simulink model "Model_14Bus_Microgrid_R2017b"  (R2017b)
settings: Solver=ode23tb  StartTime=0.0  StopTime=0.35  MaxStep=1e-2  RelTol=1e-3
InitFcn:
  | Set_parameters_R2018
StopFcn:
  | Save_Data;
  | Graphics;
values from neighbouring files (symbols this model uses):
  Clink = Ceq*2    (= 0.217013888889)    [Set_parameters_R2017b.m]    (also in Set_parameters_R2018.m)
  dis1 = 0.15    [Set_parameters_R2017b.m]    (also in Set_parameters_R2018.m)
  dis10 = 6    [Set_parameters_R2017b.m]    (also in Set_parameters_R2018.m)
  dis11 = 3    [Set_parameters_R2017b.m]    (also in Set_parameters_R2018.m)
  dis12 = 6    [Set_parameters_R2017b.m]    (also in Set_parameters_R2018.m)
  dis13 = 3    [Set_parameters_R2017b.m]    (also in Set_parameters_R2018.m)
  dis14 = 2    [Set_parameters_R2017b.m]    (also in Set_parameters_R2018.m)
  dis2 = 0.2    [Set_parameters_R2017b.m]    (also in Set_parameters_R2018.m)
  dis3 = 0.15    [Set_parameters_R2017b.m]    (also in Set_parameters_R2018.m)
  dis4 = 0.4    [Set_parameters_R2017b.m]    (also in Set_parameters_R2018.m)
  dis5 = 0.4    [Set_parameters_R2017b.m]    (also in Set_parameters_R2018.m)
  dis6 = 0.4    [Set_parameters_R2017b.m]    (also in Set_parameters_R2018.m)
  dis7 = 0.1    [Set_parameters_R2017b.m]    (also in Set_parameters_R2018.m)
  dis8 = 2    [Set_parameters_R2017b.m]    (also in Set_parameters_R2018.m)
  dis9 = 6    [Set_parameters_R2017b.m]    (also in Set_parameters_R2018.m)
  Fc = 33 * Fnom    (= 1980)    [Set_parameters_R2017b.m]    (also in Set_parameters_R2018.m)
  Fnom = 60    [Main_DC_MG.m]    (also in Set_parameters_R2017b.m; Set_parameters_R2018.m)
  Increment_MPPT = 0.01    [Set_parameters_R2017b.m]    (also in Set_parameters_R2018.m)
  Ki_Ireg = 20    [Set_parameters_R2017b.m]    (also in Set_parameters_R2018.m)
  Ki_VDCreg = 400    [Set_parameters_R2017b.m]    (also in Set_parameters_R2018.m)
  Kp_Ireg = 0.3    [Set_parameters_R2017b.m]    (also in Set_parameters_R2018.m)
  Kp_VDCreg = 2    [Set_parameters_R2017b.m]    (also in Set_parameters_R2018.m)
  LimitL_Ireg = -1.5    [Set_parameters_R2017b.m]    (also in Set_parameters_R2018.m)
  LimitL_VDCreg = -1.5    [Set_parameters_R2017b.m]    (also in Set_parameters_R2018.m)
  Limits_MPPT = [ 583 357 ]    [Set_parameters_R2017b.m]    (also in Set_parameters_R2018.m)
  LimitU_Ireg = 1.5    [Set_parameters_R2017b.m]    (also in Set_parameters_R2018.m)
  LimitU_VDCreg = 1.5    [Set_parameters_R2017b.m]    (also in Set_parameters_R2018.m)
  P_Load_2 = S_Load_2* PF_Load_2    (= 36000)    [Set_parameters_R2017b.m]    (also in Set_parameters_R2018.m)
  P_Load_3 = S_Load_3* PF_Load_3    (= 25500)    [Set_parameters_R2017b.m]    (also in Set_parameters_R2018.m)
  Pnom = 1e6    (= 1000000)    [Set_parameters_R2017b.m]    (also in Set_parameters_R2018.m)
  Pnom_T1 = 1.5e6    (= 1500000)    [Set_parameters_R2017b.m]    (also in Set_parameters_R2018.m)
  Pnom_T2 = 1.5e6    (= 1500000)    [Set_parameters_R2017b.m]    (also in Set_parameters_R2018.m)
  Pnom_T3 = 4e6    (= 4000000)    [Set_parameters_R2017b.m]    (also in Set_parameters_R2018.m)
  Pnom_xfo = Pnom    (= 1000000)    [Set_parameters_R2017b.m]    (also in Set_parameters_R2018.m)
  Ql_Load_2 = S_Load_2 * sin(acos(PF_Load_2))    [Set_parameters_R2017b.m]    (also in Set_parameters_R2018.m)
  Ql_Load_3 = S_Load_3 * sin(acos(PF_Load_3))    [Set_parameters_R2017b.m]    (also in Set_parameters_R2018.m)
  R_Load_9 = (Vnom_prim * 1.35)^2 / P_Load_9    (= 1084.6153125)    [Set_parameters_R2017b.m]    (also in Set_parameters_R2018.m)
  R_Load_DC = Vnom_DC^2/ P_Load_DC    (= 45)    [Main_DC_MG.m]    (also in Set_parameters_R2017b.m; Set_parameters_R2018.m)
  Rl = 0.394    [Set_parameters_R2017b.m]    (also in Set_parameters_R2018.m)
  Rls = 0.198    [Set_parameters_R2017b.m]    (also in Set_parameters_R2018.m)
  Ts = Ts_Power    (= 5.05050505051e-06)    [Main_DC_MG.m]    (also in Set_parameters_R2017b.m; Set_parameters_R2018.m)
  Ts_Control = 10*Ts_Power    (= 5.05050505051e-05)    [Main_DC_MG.m]    (also in Set_parameters_R2017b.m; Set_parameters_R2018.m)
  Ts_Power = 1/(33*Fnom)/100    (= 5.05050505051e-06)    [Main_DC_MG.m]    (also in Set_parameters_R2017b.m; Set_parameters_R2018.m)
  V1_LL_T3 = 69e3    (= 69000)    [Set_parameters_R2017b.m]    (also in Set_parameters_R2018.m)
  Vf = 0    [Set_parameters_R2017b.m]    (also in Set_parameters_R2018.m)
  Vfd = 0    [Set_parameters_R2017b.m]    (also in Set_parameters_R2018.m)
  Vnom_DC = 300    [Main_DC_MG.m]    (also in Set_parameters_R2017b.m; Set_parameters_R2018.m)
  Vnom_dc = 480    [Set_parameters_R2017b.m]    (also in Set_parameters_R2018.m)
  Vnom_Diesel = 2.4e3    (= 2400)    [Set_parameters_R2017b.m]    (also in Set_parameters_R2018.m)
  Vnom_prim = 13.8e3    (= 13800)    [Set_parameters_R2017b.m]    (also in Set_parameters_R2018.m)
  Vnom_sec = 220    [Set_parameters_R2017b.m]    (also in Set_parameters_R2018.m)
  Vnom_ter_AC_DC = 150    [Set_parameters_R2017b.m]    (also in Set_parameters_R2018.m)
  Xl = 0.1168    [Set_parameters_R2017b.m]    (also in Set_parameters_R2018.m)
  Xls = 0.1089    [Set_parameters_R2017b.m]    (also in Set_parameters_R2018.m)
undefined symbols (not defined in the file or in its folder): D1, Delta, Hydride, Ion, Lithium, max_min, Metal, Nickel, RL, RLff, sigbuilder_block
libraries: powerlib x202, powerlib_meascontrol x152, simulink x14, powerlib_extras x14, electricdrivelib x4, re_lib x2
(part 9 of 10)

== system Model_14Bus_Microgrid_R2017b/Bus_AC PV /PLL/Pll3 ==
  note: error
  note: d'
  note: Fundamental
  note: fase
      | total
  note: fase de la señal
  note: adelanta 90
  note: Este PLL calcula la fase respecto a una onda coseno
  señal : Inport
  w : Inport  Port=2
  Gain : Gain  Gain=-1  SaturateOnIntegerOverflow=on  OutDataTypeStr=Inherit: Same as input  ParamDataTypeStr=Inherit: Same as input
  Integrator : Integrator  InitialCondition=2*pi*60
  Integrator1 : Integrator  InitialCondition=2*pi*60
  Integrator2 : Integrator
  K : Gain  Gain=100  SaturateOnIntegerOverflow=on  OutDataTypeStr=Inherit: Same as input  ParamDataTypeStr=Inherit: Same as input
  Kp : Gain  Gain=10  SaturateOnIntegerOverflow=on  OutDataTypeStr=Inherit: Same as input  ParamDataTypeStr=Inherit: Same as input
  Kp1 : Gain  Gain=10  SaturateOnIntegerOverflow=on  OutDataTypeStr=Inherit: Same as input  ParamDataTypeStr=Inherit: Same as input
  Poduct : Product  SaturateOnIntegerOverflow=on  OutDataTypeStr=Inherit: Same as first input
  Poduct1 : Product  SaturateOnIntegerOverflow=on  OutDataTypeStr=Inherit: Same as first input
  Poduct2 : Product  SaturateOnIntegerOverflow=on  OutDataTypeStr=Inherit: Same as first input
  Sum : Sum  Inputs=|+-  SaturateOnIntegerOverflow=on
  Sum1 : Sum  SaturateOnIntegerOverflow=on
  Sum2 : Sum  Inputs=|-+  SaturateOnIntegerOverflow=on
  Trigonometric Function : Trigonometry
  Trigonometric Function1 : Trigonometry  Operator=cos
  f cos (rad) : Outport
  wires:
  Sum/1 -> Poduct/1, Poduct1/1
  Poduct/1 -> Kp/1
  Kp/1 -> Kp1/1
  Poduct2/1 -> Sum/2
  Trigonometric Function1/1 -> Poduct1/2, Poduct2/1
  Poduct1/1 -> K/1
  K/1 -> Integrator2/1
  Integrator2/1 -> Poduct2/2
  Integrator/1 -> Trigonometric Function/1, Sum2/2, Trigonometric Function1/1
  Integrator1/1 -> Sum2/1
  Sum2/1 -> f cos (rad)/1
  w/1 -> Sum1/1, Integrator1/1
  Kp1/1 -> Sum1/2
  Sum1/1 -> Integrator/1
  Trigonometric Function/1 -> Gain/1
  Gain/1 -> Poduct/2
  señal/1 -> Sum/1

== system Model_14Bus_Microgrid_R2017b/Bus_AC//DC3/Battery system/Ripple Calculations ==
  Signal : Inport
  Reset : Inport  Port=2
  0 : Constant  Value=2
  1 : Constant  Value=2
  Display10 : Display
  Display2 : Display
  Mean1 : powerlib_meascontrol/Measurements/Mean  Freq=10  Vinit=0  Ts=0
      settings: SourceProductName=Simscape Electrical
  MinMax Running Resettable : simulink/Math Operations/MinMax Running Resettable  Function=max  vinit=0.0
  MinMax Running Resettable1 : simulink/Math Operations/MinMax Running Resettable  Function=min  vinit=0.0
  Product : Product
  Product1 : Product
  Sum : Sum  Inputs=|+-
  Sum1 : Sum  Inputs=|-+
  Switch1 : Switch  Criteria=u2 > Threshold
  Switch2 : Switch  Criteria=u2 > Threshold
  Switch3 : Switch  Criteria=u2 > Threshold
  Ripple in Buck : Outport
  Ripple in Boost : Outport  Port=2
  wires:
  1/1 -> Product1/2
  [I_ref] -> Switch2/2, Switch3/2
  Product1/1 -> Switch3/3
  0/1 -> Product/2
  Switch2/1 -> Ripple in Buck/1
  Switch3/1 -> Ripple in Boost/1
  Product/1 -> Switch2/1
  Signal/1 -> Mean1/1, MinMax Running Resettable1/1, MinMax Running Resettable/1
  Switch1/1 -> Sum1/2, Sum/2
  MinMax Running Resettable/1 -> Sum/1, Display2/1
  MinMax Running Resettable1/1 -> Sum1/1, Display10/1
  Sum/1 -> Product/1
  Reset/1 -> Switch1/2, MinMax Running Resettable1/2, MinMax Running Resettable/2
  Sum1/1 -> Product1/1
  Mean1/1 -> Switch1/3

== system Model_14Bus_Microgrid_R2017b/Bus_AC//DC3/PV system/Pmean ==
  Product : Product  RndMeth=Zero
  WkW : Gain  Gain=1/1000
  P : Outport
  V : Outport  Port=2
  wires:
  [Vmean_PV] -> Product/1, V/1
  Product/1 -> WkW/1
  [Imean_PV] -> Product/2
  WkW/1 -> P/1  "Pmean_PV (kW)"

== system Model_14Bus_Microgrid_R2017b/Bus_AC//DC4/PLL/Pll1 ==
  note: error
  note: d'
  note: Fundamental
  note: fase
      | total
  note: fase de la señal
  note: adelanta 90
  note: Este PLL calcula la fase respecto a una onda coseno
  señal : Inport
  w : Inport  Port=2
  Gain : Gain  Gain=-1  SaturateOnIntegerOverflow=on  OutDataTypeStr=Inherit: Same as input  ParamDataTypeStr=Inherit: Same as input
  Integrator : Integrator  InitialCondition=2*pi*60
  Integrator1 : Integrator  InitialCondition=2*pi*60
  Integrator2 : Integrator
  K : Gain  Gain=100  SaturateOnIntegerOverflow=on  OutDataTypeStr=Inherit: Same as input  ParamDataTypeStr=Inherit: Same as input
  Kp : Gain  Gain=10  SaturateOnIntegerOverflow=on  OutDataTypeStr=Inherit: Same as input  ParamDataTypeStr=Inherit: Same as input
  Kp1 : Gain  Gain=10  SaturateOnIntegerOverflow=on  OutDataTypeStr=Inherit: Same as input  ParamDataTypeStr=Inherit: Same as input
  Poduct : Product  SaturateOnIntegerOverflow=on  OutDataTypeStr=Inherit: Same as first input
  Poduct1 : Product  SaturateOnIntegerOverflow=on  OutDataTypeStr=Inherit: Same as first input
  Poduct2 : Product  SaturateOnIntegerOverflow=on  OutDataTypeStr=Inherit: Same as first input
  Sum : Sum  Inputs=|+-  SaturateOnIntegerOverflow=on
  Sum1 : Sum  SaturateOnIntegerOverflow=on
  Sum2 : Sum  Inputs=|-+  SaturateOnIntegerOverflow=on
  Trigonometric Function : Trigonometry
  Trigonometric Function1 : Trigonometry  Operator=cos
  f cos (rad) : Outport
  wires:
  Sum/1 -> Poduct/1, Poduct1/1
  Poduct/1 -> Kp/1
  Kp/1 -> Kp1/1
  Poduct2/1 -> Sum/2
  Trigonometric Function1/1 -> Poduct1/2, Poduct2/1
  Poduct1/1 -> K/1
  K/1 -> Integrator2/1
  Integrator2/1 -> Poduct2/2
  Integrator/1 -> Trigonometric Function/1, Sum2/2, Trigonometric Function1/1
  Integrator1/1 -> Sum2/1
  Sum2/1 -> f cos (rad)/1
  w/1 -> Sum1/1, Integrator1/1
  Kp1/1 -> Sum1/2
  Sum1/1 -> Integrator/1
  Trigonometric Function/1 -> Gain/1
  Gain/1 -> Poduct/2
  señal/1 -> Sum/1

== system Model_14Bus_Microgrid_R2017b/Bus_AC//DC4/PLL/Pll2 ==
  note: error
  note: d'
  note: Fundamental
  note: fase
      | total
  note: fase de la señal
  note: adelanta 90
  note: Este PLL calcula la fase respecto a una onda coseno
  señal : Inport
  w : Inport  Port=2
  Gain : Gain  Gain=-1  SaturateOnIntegerOverflow=on  OutDataTypeStr=Inherit: Same as input  ParamDataTypeStr=Inherit: Same as input
  Integrator : Integrator  InitialCondition=2*pi*60
  Integrator1 : Integrator  InitialCondition=2*pi*60
  Integrator2 : Integrator
  K : Gain  Gain=100  SaturateOnIntegerOverflow=on  OutDataTypeStr=Inherit: Same as input  ParamDataTypeStr=Inherit: Same as input
  Kp : Gain  Gain=10  SaturateOnIntegerOverflow=on  OutDataTypeStr=Inherit: Same as input  ParamDataTypeStr=Inherit: Same as input
  Kp1 : Gain  Gain=10  SaturateOnIntegerOverflow=on  OutDataTypeStr=Inherit: Same as input  ParamDataTypeStr=Inherit: Same as input
  Poduct : Product  SaturateOnIntegerOverflow=on  OutDataTypeStr=Inherit: Same as first input
  Poduct1 : Product  SaturateOnIntegerOverflow=on  OutDataTypeStr=Inherit: Same as first input
  Poduct2 : Product  SaturateOnIntegerOverflow=on  OutDataTypeStr=Inherit: Same as first input
  Sum : Sum  Inputs=|+-  SaturateOnIntegerOverflow=on
  Sum1 : Sum  SaturateOnIntegerOverflow=on
  Sum2 : Sum  Inputs=|-+  SaturateOnIntegerOverflow=on
  Trigonometric Function : Trigonometry
  Trigonometric Function1 : Trigonometry  Operator=cos
  f cos (rad) : Outport
  wires:
  Sum/1 -> Poduct/1, Poduct1/1
  Poduct/1 -> Kp/1
  Kp/1 -> Kp1/1
  Poduct2/1 -> Sum/2
  Trigonometric Function1/1 -> Poduct1/2, Poduct2/1
  Poduct1/1 -> K/1
  K/1 -> Integrator2/1
  Integrator2/1 -> Poduct2/2
  Integrator/1 -> Trigonometric Function/1, Sum2/2, Trigonometric Function1/1
  Integrator1/1 -> Sum2/1
  Sum2/1 -> f cos (rad)/1
  w/1 -> Sum1/1, Integrator1/1
  Kp1/1 -> Sum1/2
  Sum1/1 -> Integrator/1
  Trigonometric Function/1 -> Gain/1
  Gain/1 -> Poduct/2
  señal/1 -> Sum/1

== system Model_14Bus_Microgrid_R2017b/Bus_AC//DC4/PLL/Pll3 ==
  note: error
  note: d'
  note: Fundamental
  note: fase
      | total
  note: fase de la señal
  note: adelanta 90
  note: Este PLL calcula la fase respecto a una onda coseno
  señal : Inport
  w : Inport  Port=2
  Gain : Gain  Gain=-1  SaturateOnIntegerOverflow=on  OutDataTypeStr=Inherit: Same as input  ParamDataTypeStr=Inherit: Same as input
  Integrator : Integrator  InitialCondition=2*pi*60
  Integrator1 : Integrator  InitialCondition=2*pi*60
  Integrator2 : Integrator
  K : Gain  Gain=100  SaturateOnIntegerOverflow=on  OutDataTypeStr=Inherit: Same as input  ParamDataTypeStr=Inherit: Same as input
  Kp : Gain  Gain=10  SaturateOnIntegerOverflow=on  OutDataTypeStr=Inherit: Same as input  ParamDataTypeStr=Inherit: Same as input
  Kp1 : Gain  Gain=10  SaturateOnIntegerOverflow=on  OutDataTypeStr=Inherit: Same as input  ParamDataTypeStr=Inherit: Same as input
  Poduct : Product  SaturateOnIntegerOverflow=on  OutDataTypeStr=Inherit: Same as first input
  Poduct1 : Product  SaturateOnIntegerOverflow=on  OutDataTypeStr=Inherit: Same as first input
  Poduct2 : Product  SaturateOnIntegerOverflow=on  OutDataTypeStr=Inherit: Same as first input
  Sum : Sum  Inputs=|+-  SaturateOnIntegerOverflow=on
  Sum1 : Sum  SaturateOnIntegerOverflow=on
  Sum2 : Sum  Inputs=|-+  SaturateOnIntegerOverflow=on
  Trigonometric Function : Trigonometry
  Trigonometric Function1 : Trigonometry  Operator=cos
  f cos (rad) : Outport
  wires:
  Sum/1 -> Poduct/1, Poduct1/1
  Poduct/1 -> Kp/1
  Kp/1 -> Kp1/1
  Poduct2/1 -> Sum/2
  Trigonometric Function1/1 -> Poduct1/2, Poduct2/1
  Poduct1/1 -> K/1
  K/1 -> Integrator2/1
  Integrator2/1 -> Poduct2/2
  Integrator/1 -> Trigonometric Function/1, Sum2/2, Trigonometric Function1/1
  Integrator1/1 -> Sum2/1
  Sum2/1 -> f cos (rad)/1
  w/1 -> Sum1/1, Integrator1/1
  Kp1/1 -> Sum1/2
  Sum1/1 -> Integrator/1
  Trigonometric Function/1 -> Gain/1
  Gain/1 -> Poduct/2
  señal/1 -> Sum/1

== system Model_14Bus_Microgrid_R2017b/Bus_AC//DC5/PLL/Pll1 ==
  note: error
  note: d'
  note: Fundamental
  note: fase
      | total
  note: fase de la señal
  note: adelanta 90
  note: Este PLL calcula la fase respecto a una onda coseno
  señal : Inport
  w : Inport  Port=2
  Gain : Gain  Gain=-1  SaturateOnIntegerOverflow=on  OutDataTypeStr=Inherit: Same as input  ParamDataTypeStr=Inherit: Same as input
  Integrator : Integrator  InitialCondition=2*pi*60
  Integrator1 : Integrator  InitialCondition=2*pi*60
  Integrator2 : Integrator
  K : Gain  Gain=100  SaturateOnIntegerOverflow=on  OutDataTypeStr=Inherit: Same as input  ParamDataTypeStr=Inherit: Same as input
  Kp : Gain  Gain=10  SaturateOnIntegerOverflow=on  OutDataTypeStr=Inherit: Same as input  ParamDataTypeStr=Inherit: Same as input
  Kp1 : Gain  Gain=10  SaturateOnIntegerOverflow=on  OutDataTypeStr=Inherit: Same as input  ParamDataTypeStr=Inherit: Same as input
  Poduct : Product  SaturateOnIntegerOverflow=on  OutDataTypeStr=Inherit: Same as first input
  Poduct1 : Product  SaturateOnIntegerOverflow=on  OutDataTypeStr=Inherit: Same as first input
  Poduct2 : Product  SaturateOnIntegerOverflow=on  OutDataTypeStr=Inherit: Same as first input
  Sum : Sum  Inputs=|+-  SaturateOnIntegerOverflow=on
  Sum1 : Sum  SaturateOnIntegerOverflow=on
  Sum2 : Sum  Inputs=|-+  SaturateOnIntegerOverflow=on
  Trigonometric Function : Trigonometry
  Trigonometric Function1 : Trigonometry  Operator=cos
  f cos (rad) : Outport
  wires:
  Sum/1 -> Poduct/1, Poduct1/1
  Poduct/1 -> Kp/1
  Kp/1 -> Kp1/1
  Poduct2/1 -> Sum/2
  Trigonometric Function1/1 -> Poduct1/2, Poduct2/1
  Poduct1/1 -> K/1
  K/1 -> Integrator2/1
  Integrator2/1 -> Poduct2/2
  Integrator/1 -> Trigonometric Function/1, Sum2/2, Trigonometric Function1/1
  Integrator1/1 -> Sum2/1
  Sum2/1 -> f cos (rad)/1
  w/1 -> Sum1/1, Integrator1/1
  Kp1/1 -> Sum1/2
  Sum1/1 -> Integrator/1
  Trigonometric Function/1 -> Gain/1
  Gain/1 -> Poduct/2
  señal/1 -> Sum/1

== system Model_14Bus_Microgrid_R2017b/Bus_AC//DC5/PLL/Pll2 ==
  note: error
  note: d'
  note: Fundamental
  note: fase
      | total
  note: fase de la señal
  note: adelanta 90
  note: Este PLL calcula la fase respecto a una onda coseno
  señal : Inport
  w : Inport  Port=2
  Gain : Gain  Gain=-1  SaturateOnIntegerOverflow=on  OutDataTypeStr=Inherit: Same as input  ParamDataTypeStr=Inherit: Same as input
  Integrator : Integrator  InitialCondition=2*pi*60
  Integrator1 : Integrator  InitialCondition=2*pi*60
  Integrator2 : Integrator
  K : Gain  Gain=100  SaturateOnIntegerOverflow=on  OutDataTypeStr=Inherit: Same as input  ParamDataTypeStr=Inherit: Same as input
  Kp : Gain  Gain=10  SaturateOnIntegerOverflow=on  OutDataTypeStr=Inherit: Same as input  ParamDataTypeStr=Inherit: Same as input
  Kp1 : Gain  Gain=10  SaturateOnIntegerOverflow=on  OutDataTypeStr=Inherit: Same as input  ParamDataTypeStr=Inherit: Same as input
  Poduct : Product  SaturateOnIntegerOverflow=on  OutDataTypeStr=Inherit: Same as first input
  Poduct1 : Product  SaturateOnIntegerOverflow=on  OutDataTypeStr=Inherit: Same as first input
  Poduct2 : Product  SaturateOnIntegerOverflow=on  OutDataTypeStr=Inherit: Same as first input
  Sum : Sum  Inputs=|+-  SaturateOnIntegerOverflow=on
  Sum1 : Sum  SaturateOnIntegerOverflow=on
  Sum2 : Sum  Inputs=|-+  SaturateOnIntegerOverflow=on
  Trigonometric Function : Trigonometry
  Trigonometric Function1 : Trigonometry  Operator=cos
  f cos (rad) : Outport
  wires:
  Sum/1 -> Poduct/1, Poduct1/1
  Poduct/1 -> Kp/1
  Kp/1 -> Kp1/1
  Poduct2/1 -> Sum/2
  Trigonometric Function1/1 -> Poduct1/2, Poduct2/1
  Poduct1/1 -> K/1
  K/1 -> Integrator2/1
  Integrator2/1 -> Poduct2/2
  Integrator/1 -> Trigonometric Function/1, Sum2/2, Trigonometric Function1/1
  Integrator1/1 -> Sum2/1
  Sum2/1 -> f cos (rad)/1
  w/1 -> Sum1/1, Integrator1/1
  Kp1/1 -> Sum1/2
  Sum1/1 -> Integrator/1
  Trigonometric Function/1 -> Gain/1
  Gain/1 -> Poduct/2
  señal/1 -> Sum/1

== system Model_14Bus_Microgrid_R2017b/Bus_AC//DC5/PLL/Pll3 ==
  note: error
  note: d'
  note: Fundamental
  note: fase
      | total
  note: fase de la señal
  note: adelanta 90
  note: Este PLL calcula la fase respecto a una onda coseno
  señal : Inport
  w : Inport  Port=2
  Gain : Gain  Gain=-1  SaturateOnIntegerOverflow=on  OutDataTypeStr=Inherit: Same as input  ParamDataTypeStr=Inherit: Same as input
  Integrator : Integrator  InitialCondition=2*pi*60
  Integrator1 : Integrator  InitialCondition=2*pi*60
  Integrator2 : Integrator
  K : Gain  Gain=100  SaturateOnIntegerOverflow=on  OutDataTypeStr=Inherit: Same as input  ParamDataTypeStr=Inherit: Same as input
  Kp : Gain  Gain=10  SaturateOnIntegerOverflow=on  OutDataTypeStr=Inherit: Same as input  ParamDataTypeStr=Inherit: Same as input
  Kp1 : Gain  Gain=10  SaturateOnIntegerOverflow=on  OutDataTypeStr=Inherit: Same as input  ParamDataTypeStr=Inherit: Same as input
  Poduct : Product  SaturateOnIntegerOverflow=on  OutDataTypeStr=Inherit: Same as first input
  Poduct1 : Product  SaturateOnIntegerOverflow=on  OutDataTypeStr=Inherit: Same as first input
  Poduct2 : Product  SaturateOnIntegerOverflow=on  OutDataTypeStr=Inherit: Same as first input
  Sum : Sum  Inputs=|+-  SaturateOnIntegerOverflow=on
  Sum1 : Sum  SaturateOnIntegerOverflow=on
  Sum2 : Sum  Inputs=|-+  SaturateOnIntegerOverflow=on
  Trigonometric Function : Trigonometry
  Trigonometric Function1 : Trigonometry  Operator=cos
  f cos (rad) : Outport
  wires:
  Sum/1 -> Poduct/1, Poduct1/1
  Poduct/1 -> Kp/1
  Kp/1 -> Kp1/1
  Poduct2/1 -> Sum/2
  Trigonometric Function1/1 -> Poduct1/2, Poduct2/1
  Poduct1/1 -> K/1
  K/1 -> Integrator2/1
  Integrator2/1 -> Poduct2/2
  Integrator/1 -> Trigonometric Function/1, Sum2/2, Trigonometric Function1/1
  Integrator1/1 -> Sum2/1
  Sum2/1 -> f cos (rad)/1
  w/1 -> Sum1/1, Integrator1/1
  Kp1/1 -> Sum1/2
  Sum1/1 -> Integrator/1
  Trigonometric Function/1 -> Gain/1
  Gain/1 -> Poduct/2
  señal/1 -> Sum/1

== system Model_14Bus_Microgrid_R2017b/Bus_slack /PLL/Pll1 ==
  note: error
  note: d'
  note: Fundamental
  note: fase
      | total
  note: fase de la señal
  note: adelanta 90
  note: Este PLL calcula la fase respecto a una onda coseno
  señal : Inport
  w : Inport  Port=2
  Gain : Gain  Gain=-1  SaturateOnIntegerOverflow=on  OutDataTypeStr=Inherit: Same as input  ParamDataTypeStr=Inherit: Same as input
  Integrator : Integrator  InitialCondition=2*pi*60
  Integrator1 : Integrator  InitialCondition=2*pi*60
  Integrator2 : Integrator
  K : Gain  Gain=100  SaturateOnIntegerOverflow=on  OutDataTypeStr=Inherit: Same as input  ParamDataTypeStr=Inherit: Same as input
  Kp : Gain  Gain=10  SaturateOnIntegerOverflow=on  OutDataTypeStr=Inherit: Same as input  ParamDataTypeStr=Inherit: Same as input
  Kp1 : Gain  Gain=10  SaturateOnIntegerOverflow=on  OutDataTypeStr=Inherit: Same as input  ParamDataTypeStr=Inherit: Same as input
  Poduct : Product  SaturateOnIntegerOverflow=on  OutDataTypeStr=Inherit: Same as first input
  Poduct1 : Product  SaturateOnIntegerOverflow=on  OutDataTypeStr=Inherit: Same as first input
  Poduct2 : Product  SaturateOnIntegerOverflow=on  OutDataTypeStr=Inherit: Same as first input
  Sum : Sum  Inputs=|+-  SaturateOnIntegerOverflow=on
  Sum1 : Sum  SaturateOnIntegerOverflow=on
  Sum2 : Sum  Inputs=|-+  SaturateOnIntegerOverflow=on
  Trigonometric Function : Trigonometry
  Trigonometric Function1 : Trigonometry  Operator=cos
  f cos (rad) : Outport
  wires:
  Sum/1 -> Poduct/1, Poduct1/1
  Poduct/1 -> Kp/1
  Kp/1 -> Kp1/1
  Poduct2/1 -> Sum/2
  Trigonometric Function1/1 -> Poduct1/2, Poduct2/1
  Poduct1/1 -> K/1
  K/1 -> Integrator2/1
  Integrator2/1 -> Poduct2/2
  Integrator/1 -> Trigonometric Function/1, Sum2/2, Trigonometric Function1/1
  Integrator1/1 -> Sum2/1
  Sum2/1 -> f cos (rad)/1
  w/1 -> Sum1/1, Integrator1/1
  Kp1/1 -> Sum1/2
  Sum1/1 -> Integrator/1
  Trigonometric Function/1 -> Gain/1
  Gain/1 -> Poduct/2
  señal/1 -> Sum/1

== system Model_14Bus_Microgrid_R2017b/Bus_slack /PLL/Pll2 ==
  note: error
  note: d'
  note: Fundamental
  note: fase
      | total
  note: fase de la señal
  note: adelanta 90
  note: Este PLL calcula la fase respecto a una onda coseno
  señal : Inport
  w : Inport  Port=2
  Gain : Gain  Gain=-1  SaturateOnIntegerOverflow=on  OutDataTypeStr=Inherit: Same as input  ParamDataTypeStr=Inherit: Same as input
  Integrator : Integrator  InitialCondition=2*pi*60
  Integrator1 : Integrator  InitialCondition=2*pi*60
  Integrator2 : Integrator
  K : Gain  Gain=100  SaturateOnIntegerOverflow=on  OutDataTypeStr=Inherit: Same as input  ParamDataTypeStr=Inherit: Same as input
  Kp : Gain  Gain=10  SaturateOnIntegerOverflow=on  OutDataTypeStr=Inherit: Same as input  ParamDataTypeStr=Inherit: Same as input
  Kp1 : Gain  Gain=10  SaturateOnIntegerOverflow=on  OutDataTypeStr=Inherit: Same as input  ParamDataTypeStr=Inherit: Same as input
  Poduct : Product  SaturateOnIntegerOverflow=on  OutDataTypeStr=Inherit: Same as first input
  Poduct1 : Product  SaturateOnIntegerOverflow=on  OutDataTypeStr=Inherit: Same as first input
  Poduct2 : Product  SaturateOnIntegerOverflow=on  OutDataTypeStr=Inherit: Same as first input
  Sum : Sum  Inputs=|+-  SaturateOnIntegerOverflow=on
  Sum1 : Sum  SaturateOnIntegerOverflow=on
  Sum2 : Sum  Inputs=|-+  SaturateOnIntegerOverflow=on
  Trigonometric Function : Trigonometry
  Trigonometric Function1 : Trigonometry  Operator=cos
  f cos (rad) : Outport
  wires:
  Sum/1 -> Poduct/1, Poduct1/1
  Poduct/1 -> Kp/1
  Kp/1 -> Kp1/1
  Poduct2/1 -> Sum/2
  Trigonometric Function1/1 -> Poduct1/2, Poduct2/1
  Poduct1/1 -> K/1
  K/1 -> Integrator2/1
  Integrator2/1 -> Poduct2/2
  Integrator/1 -> Trigonometric Function/1, Sum2/2, Trigonometric Function1/1
  Integrator1/1 -> Sum2/1
  Sum2/1 -> f cos (rad)/1
  w/1 -> Sum1/1, Integrator1/1
  Kp1/1 -> Sum1/2
  Sum1/1 -> Integrator/1
  Trigonometric Function/1 -> Gain/1
  Gain/1 -> Poduct/2
  señal/1 -> Sum/1

== system Model_14Bus_Microgrid_R2017b/Bus_slack /PLL/Pll3 ==
  note: error
  note: d'
  note: Fundamental
  note: fase
      | total
  note: fase de la señal
  note: adelanta 90
  note: Este PLL calcula la fase respecto a una onda coseno
  señal : Inport
  w : Inport  Port=2
  Gain : Gain  Gain=-1  SaturateOnIntegerOverflow=on  OutDataTypeStr=Inherit: Same as input  ParamDataTypeStr=Inherit: Same as input
  Integrator : Integrator  InitialCondition=2*pi*60
  Integrator1 : Integrator  InitialCondition=2*pi*60
  Integrator2 : Integrator
  K : Gain  Gain=100  SaturateOnIntegerOverflow=on  OutDataTypeStr=Inherit: Same as input  ParamDataTypeStr=Inherit: Same as input
  Kp : Gain  Gain=10  SaturateOnIntegerOverflow=on  OutDataTypeStr=Inherit: Same as input  ParamDataTypeStr=Inherit: Same as input
  Kp1 : Gain  Gain=10  SaturateOnIntegerOverflow=on  OutDataTypeStr=Inherit: Same as input  ParamDataTypeStr=Inherit: Same as input
  Poduct : Product  SaturateOnIntegerOverflow=on  OutDataTypeStr=Inherit: Same as first input
  Poduct1 : Product  SaturateOnIntegerOverflow=on  OutDataTypeStr=Inherit: Same as first input
  Poduct2 : Product  SaturateOnIntegerOverflow=on  OutDataTypeStr=Inherit: Same as first input
  Sum : Sum  Inputs=|+-  SaturateOnIntegerOverflow=on
  Sum1 : Sum  SaturateOnIntegerOverflow=on
  Sum2 : Sum  Inputs=|-+  SaturateOnIntegerOverflow=on
  Trigonometric Function : Trigonometry
  Trigonometric Function1 : Trigonometry  Operator=cos
  f cos (rad) : Outport
  wires:
  Sum/1 -> Poduct/1, Poduct1/1
  Poduct/1 -> Kp/1
  Kp/1 -> Kp1/1
  Poduct2/1 -> Sum/2
  Trigonometric Function1/1 -> Poduct1/2, Poduct2/1
  Poduct1/1 -> K/1
  K/1 -> Integrator2/1
  Integrator2/1 -> Poduct2/2
  Integrator/1 -> Trigonometric Function/1, Sum2/2, Trigonometric Function1/1
  Integrator1/1 -> Sum2/1
  Sum2/1 -> f cos (rad)/1
  w/1 -> Sum1/1, Integrator1/1
  Kp1/1 -> Sum1/2
  Sum1/1 -> Integrator/1
  Trigonometric Function/1 -> Gain/1
  Gain/1 -> Poduct/2
  señal/1 -> Sum/1

== system Model_14Bus_Microgrid_R2017b/Grid Bi-directional converter AC //CD 2 Cascaded Topology/BESS Control (A)/Subsystem ==
  Repeating Sequence : simulink/Sources/Repeating Sequence  rep_seq_t=[0 .0001 .0002 .0003 .0004 ]  rep_seq_y=[0 5 0 -5 0]
  Repeating Sequence1 : simulink/Sources/Repeating Sequence  Commented=on  rep_seq_t=[0 .0001 .0002 .0003 .0004 ]  rep_seq_y=[0 5 0 -5 0]
  Transport Delay3 : TransportDelay  Commented=on  DelayTime=.0001
  carrier : Outport
  delayed carrier : Outport  Port=2
  wires:
  Repeating Sequence/1 -> carrier/1
  Transport Delay3/1 -> delayed carrier/1
  Repeating Sequence1/1 -> Transport Delay3/1

== system Model_14Bus_Microgrid_R2017b/Grid Bi-directional converter AC //CD 2 Cascaded Topology/BESS Control (A)/Subsystem1 ==
  Constant1 : Constant  Value=max_min
  Constant2 : Constant  Value=0
  Constant3 : Constant  Value=max_min
  Gain : Gain  Gain=pi / 180 /377
  Gain1 : Gain  Gain=5
  OP_max1 : Constant  Value=216
  OP_max2 : Constant  Value=1.2
  OP_min1 : Constant  Value=252
  OP_min2 : Constant  Value=0.8
  Product1 : Product  RndMeth=Zero
  Sine Wave1 : Sin  Frequency=2*pi*Fnom  Phase=0*3.1459/180  SampleTime=0
  Sum1 : Sum  Inputs=|-+
  Switch1 : Switch  Criteria=u2 > Threshold
  Switch2 : Switch  Criteria=u2 > Threshold
  Variable Time Delay : VariableTransportDelay  MaximumDelay=16.6
  5*sin : Outport
  -5*sin : Outport  Port=2
  wires:
  Constant2/1 -> Sum1/2
  Product1/1 -> 5*sin/1, Sum1/1
  Sum1/1 -> -5*sin/1
  Switch1/1 -> Gain1/1
  Switch2/1 -> Gain/1
  Gain/1 -> Variable Time Delay/2
  Variable Time Delay/1 -> Product1/2
  Sine Wave1/1 -> Variable Time Delay/1
  Gain1/1 -> Product1/1
  OP_min1/1 -> Switch2/3
  OP_max1/1 -> Switch2/1
  Constant1/1 -> Switch2/2
  Constant3/1 -> Switch1/2
  OP_max2/1 -> Switch1/1
  OP_min2/1 -> Switch1/3

== system Model_14Bus_Microgrid_R2017b/Grid Bi-directional converter AC //CD 2 Cascaded Topology/BESS Control (B)/Subsystem2 ==
  Repeating Sequence : simulink/Sources/Repeating Sequence  rep_seq_t=[0 .0001 .0002 .0003 .0004 ]  rep_seq_y=[0 5 0 -5 0]
  Repeating Sequence1 : simulink/Sources/Repeating Sequence  Commented=on  rep_seq_t=[0 .0001 .0002 .0003 .0004 ]  rep_seq_y=[0 5 0 -5 0]
  Transport Delay1 : TransportDelay  Commented=on  DelayTime=.002333334
  Transport Delay3 : TransportDelay  DelayTime=.001333333
  carrier : Outport
  delayed carrier : Outport  Port=2
  wires:
  Repeating Sequence/1 -> Transport Delay3/1
  Transport Delay3/1 -> carrier/1
  Repeating Sequence1/1 -> Transport Delay1/1
  Transport Delay1/1 -> delayed carrier/1

== system Model_14Bus_Microgrid_R2017b/Grid Bi-directional converter AC //CD 2 Cascaded Topology/BESS Control (B)/Subsystem3 ==
  Constant1 : Constant  Value=max_min
  Constant2 : Constant  Value=0
  Constant3 : Constant  Value=max_min
  Gain : Gain  Gain=pi / 180 /377
  Gain1 : Gain  Gain=5
  OP_max1 : Constant  Value=216
  OP_max2 : Constant  Value=1.2
  OP_min1 : Constant  Value=252
  OP_min2 : Constant  Value=0.8
  Product1 : Product  RndMeth=Zero
  Sine Wave1 : Sin  Frequency=2*pi*Fnom  Phase=0*3.1459/180 - 2*pi/3  SampleTime=0
  Sum1 : Sum  Inputs=|-+
  Switch1 : Switch  Criteria=u2 > Threshold
  Switch2 : Switch  Criteria=u2 > Threshold
  Variable Time Delay : VariableTransportDelay  MaximumDelay=16.6
  4.8*sin : Outport
  -4.8*sin : Outport  Port=2
  wires:
  Sum1/1 -> -4.8*sin/1
  Product1/1 -> Sum1/1, 4.8*sin/1
  Constant2/1 -> Sum1/2
  Switch1/1 -> Gain1/1
  Gain/1 -> Variable Time Delay/2
  Sine Wave1/1 -> Variable Time Delay/1
  Variable Time Delay/1 -> Product1/2
  Switch2/1 -> Gain/1
  Gain1/1 -> Product1/1
  OP_max2/1 -> Switch1/1
  OP_min1/1 -> Switch2/3
  Constant1/1 -> Switch2/2
  OP_max1/1 -> Switch2/1
  OP_min2/1 -> Switch1/3
  Constant3/1 -> Switch1/2

== system Model_14Bus_Microgrid_R2017b/Grid Bi-directional converter AC //CD 2 Cascaded Topology/BESS Control (C)/Subsystem4 ==
  Repeating Sequence : simulink/Sources/Repeating Sequence  rep_seq_t=[0 .0001 .0002 .0003 .0004 ]  rep_seq_y=[0 5 0 -5 0]
  Repeating Sequence1 : simulink/Sources/Repeating Sequence  Commented=on  rep_seq_t=[0 .0001 .0002 .0003 .0004 ]  rep_seq_y=[0 5 0 -5 0]
  Transport Delay1 : TransportDelay  DelayTime=.002666667
  Transport Delay3 : TransportDelay  Commented=on  DelayTime=.003444444
  carrier : Outport
  delayed carrier : Outport  Port=2
  wires:
  Transport Delay3/1 -> delayed carrier/1
  Repeating Sequence1/1 -> Transport Delay3/1
  Repeating Sequence/1 -> Transport Delay1/1
  Transport Delay1/1 -> carrier/1

== system Model_14Bus_Microgrid_R2017b/Grid Bi-directional converter AC //CD 2 Cascaded Topology/BESS Control (C)/Subsystem5 ==
  Constant1 : Constant  Value=max_min
  Constant2 : Constant  Value=0
  Constant3 : Constant  Value=max_min
  Gain : Gain  Gain=pi / 180 /377
  Gain1 : Gain  Gain=5
  OP_max1 : Constant  Value=216
  OP_max2 : Constant  Value=1.2
  OP_min1 : Constant  Value=252
  OP_min2 : Constant  Value=0.8
  Product1 : Product  RndMeth=Zero
  Sine Wave1 : Sin  Frequency=2*pi*Fnom  Phase=0*3.1459/180 + 2*pi/3  SampleTime=0
  Sum1 : Sum  Inputs=|-+
  Switch1 : Switch  Criteria=u2 > Threshold
  Switch2 : Switch  Criteria=u2 > Threshold
  Variable Time Delay : VariableTransportDelay  MaximumDelay=16.6
  4.8*sin : Outport
  -4.8*sin : Outport  Port=2
  wires:
  Constant2/1 -> Sum1/2
  Product1/1 -> 4.8*sin/1, Sum1/1
  Sum1/1 -> -4.8*sin/1
  Sine Wave1/1 -> Variable Time Delay/1
  Gain/1 -> Variable Time Delay/2
  Variable Time Delay/1 -> Product1/2
  Switch1/1 -> Gain1/1
  Gain1/1 -> Product1/1
  Switch2/1 -> Gain/1
  OP_max2/1 -> Switch1/1
  OP_min1/1 -> Switch2/3
  Constant1/1 -> Switch2/2
  OP_max1/1 -> Switch2/1
  OP_min2/1 -> Switch1/3
  Constant3/1 -> Switch1/2

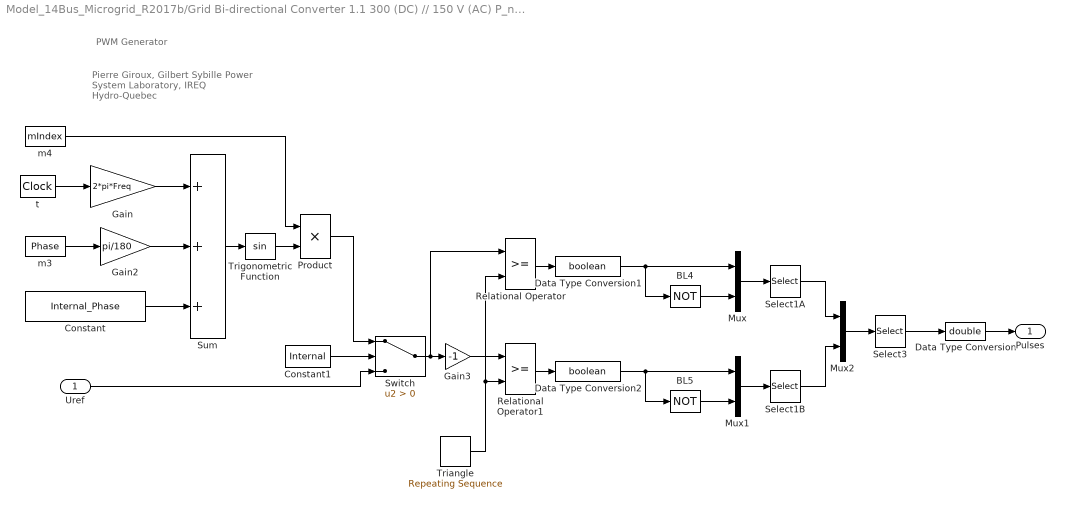
== system Model_14Bus_Microgrid_R2017b/Grid Bi-directional Converter 1.1 300 (DC) // 150 V (AC) P_nom 3kW/Control of Inverter/Discrete PWM Generator1 ==
  note: Pierre Giroux, Gilbert Sybille
      | Power System Laboratory, IREQ
      | Hydro-Quebec
  note: PWM Generator
  Uref : Inport
  BL4 : Logic  Operator=NOT  Inputs=1
  BL5 : Logic  Operator=NOT  Inputs=1
  Constant : Constant  Value=Internal_Phase
  Constant1 : Constant  Value=Internal
  Data Type Conversion : DataTypeConversion  OutDataTypeStr=double  SaturateOnIntegerOverflow=on  RndMeth=Zero
  Data Type Conversion1 : DataTypeConversion  OutDataTypeStr=boolean  SaturateOnIntegerOverflow=on  RndMeth=Zero
  Data Type Conversion2 : DataTypeConversion  OutDataTypeStr=boolean  SaturateOnIntegerOverflow=on  RndMeth=Zero
  Gain : Gain  Gain=2*pi*Freq  SaturateOnIntegerOverflow=on  OutDataTypeStr=Inherit: Same as input  ParamDataTypeStr=Inherit: Same as input
  Gain2 : Gain  Gain=pi/180  SaturateOnIntegerOverflow=on  OutDataTypeStr=Inherit: Same as input  ParamDataTypeStr=Inherit: Same as input
  Gain3 : Gain  Gain=-1  SaturateOnIntegerOverflow=on  OutDataTypeStr=Inherit: Same as input  ParamDataTypeStr=Inherit: Same as input
  Mux : Mux  Inputs=2
  Mux1 : Mux  Inputs=2
  Mux2 : Mux  Inputs=2
  Product : Product  SaturateOnIntegerOverflow=on  InputSameDT=on  OutDataTypeStr=Inherit: Same as first input
  Relational Operator : RelationalOperator  RndMeth=Nearest  InputSameDT=on
  Relational Operator1 : RelationalOperator  RndMeth=Nearest  InputSameDT=on
  Select1A : Selector  InputPortWidth=Select1_PortWidth  IndexOptions=Index vector (dialog)  Indices=Select1_Elements  OutputSizes=1
  Select1B : Selector  InputPortWidth=Select1_PortWidth  IndexOptions=Index vector (dialog)  Indices=Select1_Elements  OutputSizes=1
  Select3 : Selector  InputPortWidth=Select3_PortWidth  IndexOptions=Index vector (dialog)  Indices=Select3_Elements  OutputSizes=1
  Sum : Sum  Inputs=+++  SaturateOnIntegerOverflow=on  InputSameDT=on  OutDataTypeStr=Inherit: Same as first input
  Switch : Switch  Criteria=u2 > Threshold
  Triangle : simulink/Sources/Repeating Sequence  rep_seq_t=[0 1/Fc/4 3/Fc/4 1/Fc]  rep_seq_y=[0 -1 1 0]
  Trigonometric Function : Trigonometry
  m3 : Constant  Value=Phase
  m4 : Constant  Value=mIndex
  t : DigitalClock  SampleTime=Ts
  Pulses : Outport
  wires:
  Mux2/1 -> Select3/1
  Select1B/1 -> Mux2/2
  Select1A/1 -> Mux2/1
  Mux1/1 -> Select1B/1
  Mux/1 -> Select1A/1
  BL5/1 -> Mux1/2
  BL4/1 -> Mux/2
  Gain3/1 -> Relational Operator1/1
  Triangle/1 -> Relational Operator1/2, Relational Operator/2
  Product/1 -> Switch/1
  Constant1/1 -> Switch/2
  Trigonometric Function/1 -> Product/2
  Sum/1 -> Trigonometric Function/1
  m4/1 -> Product/1
  Constant/1 -> Sum/3
  m3/1 -> Gain2/1
  Gain2/1 -> Sum/2
  Gain/1 -> Sum/1
  t/1 -> Gain/1
  Select3/1 -> Data Type Conversion/1
  Data Type Conversion/1 -> Pulses/1
  Relational Operator/1 -> Data Type Conversion1/1
  Data Type Conversion1/1 -> BL4/1, Mux/1
  Relational Operator1/1 -> Data Type Conversion2/1
  Data Type Conversion2/1 -> BL5/1, Mux1/1
  Switch/1 -> Relational Operator/1, Gain3/1
  Uref/1 -> Switch/3

== system Model_14Bus_Microgrid_R2017b/Grid Bi-directional Converter 1.1 300 (DC) // 150 V (AC) P_nom 3kW/Control of Inverter/MI Controller ==
  Vabc : Inport
  Demux : Demux  Commented=on  Outputs=3
  Demux1 : Demux  Outputs=3
  Mux : Mux  Inputs=3
  Mux1 : Mux  Inputs=3
  Mux2 : Mux  Inputs=3
  OP max / min : Subsystem
  Product : Product  RndMeth=Zero
  Product1 : Product  RndMeth=Zero
  Product2 : Product  RndMeth=Zero
  Subsystem : Subsystem
  Subsystem1 : Subsystem
  Terminator : Terminator
  Terminator1 : Terminator  Commented=on
  Terminator2 : Terminator  Commented=on
  Terminator3 : Terminator
  Terminator4 : Terminator  Commented=on
  Vab1 : powerlib_extras/Discrete Measurements/Discrete  RMS value  Commented=on  Freq=60  Mag_Init=0  Ts=20e-6
  Vab5 : powerlib_extras/Discrete Measurements/Discrete  RMS value  Commented=on  Freq=60  Mag_Init=0  Ts=20e-6
  Vab6 : powerlib_extras/Discrete Measurements/Discrete  RMS value  Commented=on  Freq=60  Mag_Init=0  Ts=20e-6
  Vabc_inv : Outport
  u / m : Outport  Port=2
  wires:
  Product/1 -> Mux2/1
  Product1/1 -> Mux2/2
  Product2/1 -> Mux2/3
  Mux1/1 -> u / m/1
  Vabc/1 -> Demux/1
  Demux/1 -> Vab6/1
  Demux/2 -> Vab5/1
  Demux/3 -> Vab1/1
  Demux1/1 -> Product/1, Mux1/1
  Demux1/2 -> Product1/1, Mux1/2
  Demux1/3 -> Product2/1, Mux1/3
  Subsystem/1(Va) -> Product/2
  Subsystem/2(Vb) -> Product1/2
  Subsystem/3(Vc) -> Product2/2
  Mux2/1 -> Vabc_inv/1
  Vab6/1 -> Terminator2/1
  Subsystem1/3(wt) -> Terminator/1
  Subsystem1/1(Frec) -> Terminator3/1
  Subsystem1/2(sin_cos) -> Subsystem/1(sin_cos)
  Mux/1 -> Demux1/1
  OP max / min/1(ctrl) -> Mux/3, Mux/1, Mux/2
  Vab5/1 -> Terminator1/1
  Vab1/1 -> Terminator4/1

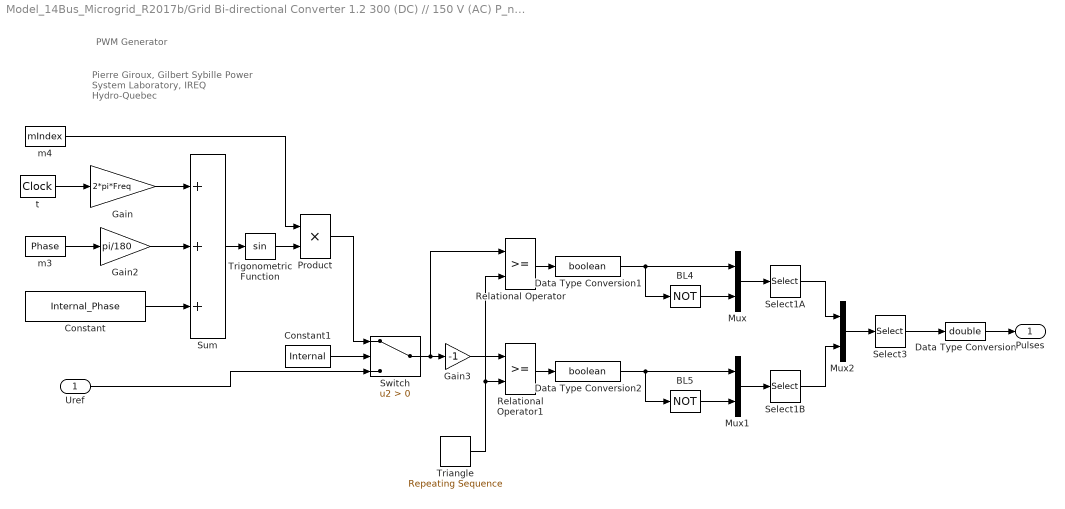
== system Model_14Bus_Microgrid_R2017b/Grid Bi-directional Converter 1.2 300 (DC) // 150 V (AC) P_nom 3kW/Control of Inverter/Discrete PWM Generator1 ==
  note: Pierre Giroux, Gilbert Sybille
      | Power System Laboratory, IREQ
      | Hydro-Quebec
  note: PWM Generator
  Uref : Inport
  BL4 : Logic  Operator=NOT  Inputs=1
  BL5 : Logic  Operator=NOT  Inputs=1
  Constant : Constant  Value=Internal_Phase
  Constant1 : Constant  Value=Internal
  Data Type Conversion : DataTypeConversion  OutDataTypeStr=double  SaturateOnIntegerOverflow=on  RndMeth=Zero
  Data Type Conversion1 : DataTypeConversion  OutDataTypeStr=boolean  SaturateOnIntegerOverflow=on  RndMeth=Zero
  Data Type Conversion2 : DataTypeConversion  OutDataTypeStr=boolean  SaturateOnIntegerOverflow=on  RndMeth=Zero
  Gain : Gain  Gain=2*pi*Freq  SaturateOnIntegerOverflow=on  OutDataTypeStr=Inherit: Same as input  ParamDataTypeStr=Inherit: Same as input
  Gain2 : Gain  Gain=pi/180  SaturateOnIntegerOverflow=on  OutDataTypeStr=Inherit: Same as input  ParamDataTypeStr=Inherit: Same as input
  Gain3 : Gain  Gain=-1  SaturateOnIntegerOverflow=on  OutDataTypeStr=Inherit: Same as input  ParamDataTypeStr=Inherit: Same as input
  Mux : Mux  Inputs=2
  Mux1 : Mux  Inputs=2
  Mux2 : Mux  Inputs=2
  Product : Product  SaturateOnIntegerOverflow=on  InputSameDT=on  OutDataTypeStr=Inherit: Same as first input
  Relational Operator : RelationalOperator  RndMeth=Nearest  InputSameDT=on
  Relational Operator1 : RelationalOperator  RndMeth=Nearest  InputSameDT=on
  Select1A : Selector  InputPortWidth=Select1_PortWidth  IndexOptions=Index vector (dialog)  Indices=Select1_Elements  OutputSizes=1
  Select1B : Selector  InputPortWidth=Select1_PortWidth  IndexOptions=Index vector (dialog)  Indices=Select1_Elements  OutputSizes=1
  Select3 : Selector  InputPortWidth=Select3_PortWidth  IndexOptions=Index vector (dialog)  Indices=Select3_Elements  OutputSizes=1
  Sum : Sum  Inputs=+++  SaturateOnIntegerOverflow=on  InputSameDT=on  OutDataTypeStr=Inherit: Same as first input
  Switch : Switch  Criteria=u2 > Threshold
  Triangle : simulink/Sources/Repeating Sequence  rep_seq_t=[0 1/Fc/4 3/Fc/4 1/Fc]  rep_seq_y=[0 -1 1 0]
  Trigonometric Function : Trigonometry
  m3 : Constant  Value=Phase
  m4 : Constant  Value=mIndex
  t : DigitalClock  SampleTime=Ts
  Pulses : Outport
  wires:
  Mux2/1 -> Select3/1
  Select1B/1 -> Mux2/2
  Select1A/1 -> Mux2/1
  Mux1/1 -> Select1B/1
  Mux/1 -> Select1A/1
  BL5/1 -> Mux1/2
  BL4/1 -> Mux/2
  Gain3/1 -> Relational Operator1/1
  Triangle/1 -> Relational Operator1/2, Relational Operator/2
  Product/1 -> Switch/1
  Constant1/1 -> Switch/2
  Trigonometric Function/1 -> Product/2
  Sum/1 -> Trigonometric Function/1
  m4/1 -> Product/1
  Constant/1 -> Sum/3
  m3/1 -> Gain2/1
  Gain2/1 -> Sum/2
  Gain/1 -> Sum/1
  t/1 -> Gain/1
  Select3/1 -> Data Type Conversion/1
  Data Type Conversion/1 -> Pulses/1
  Relational Operator/1 -> Data Type Conversion1/1
  Data Type Conversion1/1 -> BL4/1, Mux/1
  Relational Operator1/1 -> Data Type Conversion2/1
  Data Type Conversion2/1 -> BL5/1, Mux1/1
  Switch/1 -> Relational Operator/1, Gain3/1
  Uref/1 -> Switch/3

== system Model_14Bus_Microgrid_R2017b/Grid Bi-directional Converter 1.2 300 (DC) // 150 V (AC) P_nom 3kW/Control of Inverter/MI Controller ==
  Vabc : Inport
  Cd to AC : Constant  Value=1.2
  Demux : Demux  Commented=on  Outputs=3
  Demux1 : Demux  Outputs=3
  Mux : Mux  Inputs=3
  Mux1 : Mux  Inputs=3
  Mux2 : Mux  Inputs=3
  Product : Product  RndMeth=Zero
  Product1 : Product  RndMeth=Zero
  Product2 : Product  RndMeth=Zero
  Subsystem : Subsystem
  Subsystem1 : Subsystem
  Terminator1 : Terminator  Commented=on
  Terminator2 : Terminator  Commented=on
  Terminator3 : Terminator
  Terminator4 : Terminator
  Terminator5 : Terminator  Commented=on
  Vab1 : powerlib_extras/Discrete Measurements/Discrete  RMS value  Commented=on  Freq=60  Mag_Init=0  Ts=20e-6
  Vab5 : powerlib_extras/Discrete Measurements/Discrete  RMS value  Commented=on  Freq=60  Mag_Init=0  Ts=20e-6
  Vab6 : powerlib_extras/Discrete Measurements/Discrete  RMS value  Commented=on  Freq=60  Mag_Init=0  Ts=20e-6
  Vabc_inv : Outport
  m : Outport  Port=2
  wires:
  Product/1 -> Mux2/1
  Product1/1 -> Mux2/2
  Product2/1 -> Mux2/3
  Mux1/1 -> m/1
  Vabc/1 -> Demux/1
  Demux/1 -> Vab6/1
  Demux/2 -> Vab5/1
  Demux/3 -> Vab1/1
  Demux1/1 -> Product/1, Mux1/1
  Demux1/2 -> Product1/1, Mux1/2
  Demux1/3 -> Product2/1, Mux1/3
  Subsystem/1(Va) -> Product/2
  Subsystem/2(Vb) -> Product1/2
  Subsystem/3(Vc) -> Product2/2
  Mux2/1 -> Vabc_inv/1
  Vab6/1 -> Terminator2/1
  Subsystem1/3(wt) -> Terminator3/1
  Subsystem1/2(sin_cos) -> Subsystem/1(sin_cos)
  Subsystem1/1(Frec) -> Terminator4/1
  Cd to AC/1 -> Mux/1, Mux/2, Mux/3
  Mux/1 -> Demux1/1
  Vab5/1 -> Terminator1/1
  Vab1/1 -> Terminator5/1

== system Model_14Bus_Microgrid_R2017b/Grid Inverter PV 480 // 250 DC // AC /Inverter Control/Current Regulator ==
  note: Current Regulator
      | ================
  note: Sign Convention: Current going out of the converter = positive current
  note: Iq positive --> The converter absorbs reactive power ("Inductive mode") = Reactive Power Q negative
  note: Id positive --> The converter generates active power ("Inverter mode") = Active Power P positive
  VdVq_meas : Inport  PortDimensions=2
  IdIq_meas : Inport  Port=2  PortDimensions=2
  IdIq_ref : Inport  Port=3  PortDimensions=2
  Add1 : Sum  Inputs=++-
  Add2 : Sum
  Add3 : Sum  Inputs=+++
  Demux : Demux  Outputs=2
  Demux1 : Demux  Outputs=2
  Lff : Gain  Gain=RLff(2)  SaturateOnIntegerOverflow=on  OutDataTypeStr=Inherit: Same as input  ParamDataTypeStr=Inherit: Same as input
  "Lff  " : Gain  Gain=RLff(2)  SaturateOnIntegerOverflow=on  OutDataTypeStr=Inherit: Same as input  ParamDataTypeStr=Inherit: Same as input
  Mux : Mux  Inputs=2
  PI : simulink/Continuous/PID Controller  Controller=PI  Form=Parallel  TimeDomain=Discrete-time  SampleTime=Ts_Control  IntegratorMethod=Forward Euler  FilterMethod=Forward Euler  ControllerParametersSource=internal  P=Kp_Ireg  I=Ki_Ireg  D=0  UseFilter=on  N=100  TunerSelectOption=Transfer Function Based (PID Tuner App)  InitialConditionSource=internal  InitialConditionForIntegrator=0  InitialConditionForFilter=0  DifferentiatorICPrevScaledInput=0  ExternalReset=none  TrackingMode=off  Kt=1  LimitOutput=on  UpperSaturationLimit=LimitU_Ireg  LowerSaturationLimit=LimitL_Ireg  LinearizeAsGain=off  AntiWindupMode=none  Kb=1  POutMin=[]  POutMax=[]  IOutMin=[]  IOutMax=[]  DOutMin=[]  DOutMax=[]  NOutMin=[]  NOutMax=[]  SumOutMin=[]  SumOutMax=[]  SaturationOutMin=[]  SaturationOutMax=[]  PParamMin=[]  PParamMax=[]  IParamMin=[]  IParamMax=[]  DParamMin=[]  DParamMax=[]  NParamMin=[]  NParamMax=[]  KbParamMin=[]  KbParamMax=[]  KtParamMin=[]  KtParamMax=[]  KbOutMin=[]  KbOutMax=[]  KtOutMin=[]  KtOutMax=[]  IntegratorOutMin=[]  IntegratorOutMax=[]  FilterOutMin=[]  FilterOutMax=[]  SumI1OutMin=[]  SumI1OutMax=[]  SumI2OutMin=[]  SumI2OutMax=[]  SumI3OutMin=[]  SumI3OutMax=[]  SumDOutMin=[]  SumDOutMax=[]  DifferentiatorOutMin=[]  DifferentiatorOutMax=[]  FilterDiffOutCoefMin=[]  FilterDiffOutCoefMax=[]  ReciprocalOutMin=[]  ReciprocalOutMax=[]  SumDenOutMin=[]  SumDenOutMax=[]  SumNumOutMin=[]  SumNumOutMax=[]  DivideOutMin=[]  DivideOutMax=[]  IntegratorContinuousStateAttributes=''  IntegratorStateMustResolveToSignalObject=off  IntegratorRTWStateStorageClass=Auto  FilterContinuousStateAttributes=''  FilterStateMustResolveToSignalObject=off  FilterRTWStateStorageClass=Auto
  PI_Ireg1 : Scope
  Rff : Gain  Gain=RLff(1)  SaturateOnIntegerOverflow=on  OutDataTypeStr=Inherit: Same as input  ParamDataTypeStr=Inherit: Same as input
  "Rff " : Gain  Gain=RLff(1)  SaturateOnIntegerOverflow=on  OutDataTypeStr=Inherit: Same as input  ParamDataTypeStr=Inherit: Same as input
  Saturation : Saturate  UpperLimit=LimitU_Ireg  LowerLimit=LimitL_Ireg
  Sum : Sum  Inputs=|-+
  VdVq_conv : Outport
  wires:
  Mux/1 -> Add2/2
  PI/1 -> PI_Ireg1/1, Add2/1  "PI"
  Sum/1 -> PI/1
  IdIq_ref/1 -> Sum/2, Demux1/1
  IdIq_meas/1 -> Sum/1
  Add2/1 -> Saturation/1
  Saturation/1 -> VdVq_conv/1
  VdVq_meas/1 -> Demux/1
  Demux/1 -> Add1/1
  "Rff "/1 -> Add1/2
  Demux1/1 -> "Rff "/1, Lff/1
  "Lff  "/1 -> Add1/3
  Demux1/2 -> "Lff  "/1, Rff/1
  Rff/1 -> Add3/2
  Lff/1 -> Add3/3
  Add1/1 -> Mux/1  "Feedforward"
  Demux/2 -> Add3/1
  Add3/1 -> Mux/2

== system Model_14Bus_Microgrid_R2017b/Grid Inverter PV 480 // 250 DC // AC /Inverter Control/MPPT Parameters ==
  note: Parameters for Perturb and Observe Algorithm:
  note: Lower limit for Vdc_ref (Dmax)
  note: Initial value for Vdc_ref output (Dinit)
  note: Increment value used to increase/decrease Vdc_ref (DeltaD)
  note: Upper limit for Vdc_ref (Dmax)
  Iph_ : Constant  Value=Vdc_ref_Init
  Iph_1 : Constant  Value=Limits_MPPT(1)
  Iph_2 : Constant  Value=Limits_MPPT(2)
  Iph_3 : Constant  Value=Increment_MPPT
  Mux : Mux
  Param : Outport
  wires:
  Mux/1 -> Param/1
  Iph_3/1 -> Mux/4
  Iph_2/1 -> Mux/3
  Iph_1/1 -> Mux/2
  Iph_/1 -> Mux/1

== system Model_14Bus_Microgrid_R2017b/Grid Inverter PV 480 // 250 DC // AC /Inverter Control/PLL & Measurements ==
  note: PLL & Measurements
      | ===================
  Vabc_prim : Inport
  Iabc_prim : Inport  Port=2
  PLL (3ph) : powerlib_meascontrol/PLL/PLL (3ph)  Fmin=45  Par_Init="[-0.57  Fnom]"  ParK=[180, 3200, 1]  TcD=1e-4  MaxRateChangeFreq=12  FilterCutOffFreq=25  Ts=Ts_Control  AGC=on
      settings: SourceProductName=Simscape Electrical
  Selector1 : Selector  InputPortWidth=3  IndexOptions=Index vector (dialog)  Indices=[1 2]  OutputSizes=1
  Selector2 : Selector  InputPortWidth=3  IndexOptions=Index vector (dialog)  Indices=[1 2]  OutputSizes=1
  Terminator : Terminator
  V->pu : Gain  Gain=1/(Vnom_prim*sqrt(2)/sqrt(3))  SaturateOnIntegerOverflow=on  OutDataTypeStr=Inherit: Same as input  ParamDataTypeStr=Inherit: Same as input
  V->pu1 : Gain  Gain=Vnom_prim*sqrt(3)/Pnom/sqrt(2)  SaturateOnIntegerOverflow=on  OutDataTypeStr=Inherit: Same as input  ParamDataTypeStr=Inherit: Same as input
  abc to dq0 : powerlib_meascontrol/Transformations/abc to dq0  Alignment=90 degrees behind phase A axis
      settings: SourceProductName=Simscape Electrical
  abc to dq1 : powerlib_meascontrol/Transformations/abc to dq0  Alignment=90 degrees behind phase A axis
      settings: SourceProductName=Simscape Electrical
  wt : Outport
  VdVq_prim : Outport  Port=2
  IdIq_prim : Outport  Port=3
  tag scope: IdIq_prim=global
  wires:
  V->pu1/1 -> abc to dq1/1
  V->pu/1 -> PLL (3ph)/1, abc to dq0/1
  abc to dq1/1 -> Selector1/1
  Vabc_prim/1 -> V->pu/1
  Iabc_prim/1 -> V->pu1/1
  abc to dq0/1 -> Selector2/1
  Selector2/1 -> VdVq_prim/1
  Selector1/1 -> [IdIq_prim], IdIq_prim/1
  PLL (3ph)/2 -> wt/1, abc to dq1/2, abc to dq0/2
  PLL (3ph)/1 -> Terminator/1

== system Model_14Bus_Microgrid_R2017b/Grid Inverter PV 480 // 250 DC // AC /Inverter Control/Uabc_ref Generation max (m) = 1 ==
  note: (Correction for transformer
      |  D1 connection)
  note: (Correction for delai of Ts_Control)
  note: Uref Generation
      | ==============
  wt : Inport
  VdVq_conv : Inport  Port=2
  Add1 : Sum  Inputs=++++
  Add2 : Sum
  Complex to Magnitude-Angle : ComplexToMagnitudeAngle
  Constant : Constant  Value=-pi/6
  Constant1 : Constant  Value=Vnom_dc
  Constant2 : Constant  Value="[ 0  -2*pi/3  2*pi/3  ]"
  Constant3 : Constant  Value=Vnom_sec*sqrt(2)/sqrt(3)
  Constant4 : Constant  Value=Ts_Control*Fnom*(2*pi)
  Demux1 : Demux  Outputs=2
  Gain1 : Gain  Gain=1/2
  Product : Product  Inputs=*/  RndMeth=Zero
  Product1 : Product  Inputs=*/  RndMeth=Zero
  Product2 : Product  Inputs=**  RndMeth=Zero
  Real-Imag to Complex : RealImagToComplex
  Trigonometric Function : Trigonometry
  Uabc_ref : Outport
  tag scope: m=global
  wires:
  Constant1/1 -> Gain1/1
  VdVq_conv/1 -> Product1/1
  Product1/1 -> Demux1/1
  Gain1/1 -> Product/1
  Real-Imag to Complex/1 -> Complex to Magnitude-Angle/1
  Demux1/1 -> Real-Imag to Complex/1
  Demux1/2 -> Real-Imag to Complex/2
  Constant2/1 -> Add1/2
  Constant/1 -> Add1/3
  Constant3/1 -> Product/2
  Product/1 -> Product1/2
  Complex to Magnitude-Angle/2 -> Add2/1
  Add1/1 -> Add2/2
  Add2/1 -> Trigonometric Function/1
  Complex to Magnitude-Angle/1 -> [m], Product2/1
  Trigonometric Function/1 -> Product2/2
  Product2/1 -> Uabc_ref/1
  wt/1 -> Add1/1
  Constant4/1 -> Add1/4
